simulink model "ABC"  (R2016b)
settings: Solver=VariableStepAuto  StartTime=0.0  StopTime=10.0  RelTol=1e-3
model workspace (MAT data in the model file):
  ContractValidatorBlocksMap = containers.Map
  ContractValidatorBlocksMap.serialization.keys = {'ABC/S/ASpec/validator', 'ABC/S/BSpec/validator', 'ABC/S/CSpec/validator', 'ABC/S_Spec/validator', 'ABC/Subsystem/ASpec/validator', 'ABC/Subsystem/BSpec/validator', 'ABC/Subsystem/BSpec1/validator', 'ABC/contract/validator'}
  ContractValidatorBlocksMap.serialization.values{1}.block = 'ABC/S/ASpec/validator'
  ContractValidatorBlocksMap.serialization.values{1}.assumePorts = 1
  ContractValidatorBlocksMap.serialization.values{1}.guaranteePorts = 1
  ContractValidatorBlocksMap.serialization.values{1}.modeBlocksPorts = 0
  ContractValidatorBlocksMap.serialization.values{1}.portHandles.Inport = [194.002685547 195.002685547]
  ContractValidatorBlocksMap.serialization.values{1}.portHandles.Outport = 196.002685547
  ContractValidatorBlocksMap.serialization.values{1}.portHandles.Enable = []
  ContractValidatorBlocksMap.serialization.values{1}.portHandles.Trigger = []
  ContractValidatorBlocksMap.serialization.values{1}.portHandles.State = []
  ContractValidatorBlocksMap.serialization.values{1}.portHandles.LConn = []
  ContractValidatorBlocksMap.serialization.values{1}.portHandles.RConn = []
  ContractValidatorBlocksMap.serialization.values{1}.portHandles.Ifaction = []
  ContractValidatorBlocksMap.serialization.values{1}.portHandles.Reset = []
  ContractValidatorBlocksMap.serialization.values{1}.portConnectivity(1).Type = '1'
  ContractValidatorBlocksMap.serialization.values{1}.portConnectivity(1).Position = [365 -50]
  ContractValidatorBlocksMap.serialization.values{1}.portConnectivity(1).SrcBlock = 19.0026855469
  ContractValidatorBlocksMap.serialization.values{1}.portConnectivity(1).SrcPort = 0
  ContractValidatorBlocksMap.serialization.values{1}.portConnectivity(1).DstBlock = []
  ContractValidatorBlocksMap.serialization.values{1}.portConnectivity(1).DstPort = []
  ContractValidatorBlocksMap.serialization.values{1}.portConnectivity(2).Type = '2'
  ContractValidatorBlocksMap.serialization.values{1}.portConnectivity(2).Position = [365 200]
  ContractValidatorBlocksMap.serialization.values{1}.portConnectivity(2).SrcBlock = 26.0026855469
  ContractValidatorBlocksMap.serialization.values{1}.portConnectivity(2).SrcPort = 0
  ContractValidatorBlocksMap.serialization.values{1}.portConnectivity(2).DstBlock = []
  ContractValidatorBlocksMap.serialization.values{1}.portConnectivity(2).DstPort = []
  ContractValidatorBlocksMap.serialization.values{1}.portConnectivity(3).Type = '1'
  ContractValidatorBlocksMap.serialization.values{1}.portConnectivity(3).Position = [500 75]
  ContractValidatorBlocksMap.serialization.values{1}.portConnectivity(3).SrcBlock = []
  ContractValidatorBlocksMap.serialization.values{1}.portConnectivity(3).SrcPort = []
  ContractValidatorBlocksMap.serialization.values{1}.portConnectivity(3).DstBlock = 38.0026855469
  ContractValidatorBlocksMap.serialization.values{1}.portConnectivity(3).DstPort = 0
  ContractValidatorBlocksMap.serialization.values{2}.block = 'ABC/S/BSpec/validator'
  ContractValidatorBlocksMap.serialization.values{2}.assumePorts = 1
  ContractValidatorBlocksMap.serialization.values{2}.guaranteePorts = 1
  ContractValidatorBlocksMap.serialization.values{2}.modeBlocksPorts = 0
  ContractValidatorBlocksMap.serialization.values{2}.portHandles.Inport = [191.002685547 192.002685547]
  ContractValidatorBlocksMap.serialization.values{2}.portHandles.Outport = 193.002685547
  ContractValidatorBlocksMap.serialization.values{2}.portHandles.Enable = []
  ContractValidatorBlocksMap.serialization.values{2}.portHandles.Trigger = []
  ContractValidatorBlocksMap.serialization.values{2}.portHandles.State = []
  ContractValidatorBlocksMap.serialization.values{2}.portHandles.LConn = []
  ContractValidatorBlocksMap.serialization.values{2}.portHandles.RConn = []
  ContractValidatorBlocksMap.serialization.values{2}.portHandles.Ifaction = []
  ContractValidatorBlocksMap.serialization.values{2}.portHandles.Reset = []
  ContractValidatorBlocksMap.serialization.values{2}.portConnectivity(1).Type = '1'
  ContractValidatorBlocksMap.serialization.values{2}.portConnectivity(1).Position = [365 -50]
  ContractValidatorBlocksMap.serialization.values{2}.portConnectivity(1).SrcBlock = 60.0026855469
  ContractValidatorBlocksMap.serialization.values{2}.portConnectivity(1).SrcPort = 0
  ContractValidatorBlocksMap.serialization.values{2}.portConnectivity(1).DstBlock = []
  ContractValidatorBlocksMap.serialization.values{2}.portConnectivity(1).DstPort = []
  ContractValidatorBlocksMap.serialization.values{2}.portConnectivity(2).Type = '2'
  ContractValidatorBlocksMap.serialization.values{2}.portConnectivity(2).Position = [365 200]
  ContractValidatorBlocksMap.serialization.values{2}.portConnectivity(2).SrcBlock = 67.0026855469
  ContractValidatorBlocksMap.serialization.values{2}.portConnectivity(2).SrcPort = 0
  ContractValidatorBlocksMap.serialization.values{2}.portConnectivity(2).DstBlock = []
  ContractValidatorBlocksMap.serialization.values{2}.portConnectivity(2).DstPort = []
  ContractValidatorBlocksMap.serialization.values{2}.portConnectivity(3).Type = '1'
  ContractValidatorBlocksMap.serialization.values{2}.portConnectivity(3).Position = [500 75]
  ContractValidatorBlocksMap.serialization.values{2}.portConnectivity(3).SrcBlock = []
  ContractValidatorBlocksMap.serialization.values{2}.portConnectivity(3).SrcPort = []
  ContractValidatorBlocksMap.serialization.values{2}.portConnectivity(3).DstBlock = 81.0026855469
  ContractValidatorBlocksMap.serialization.values{2}.portConnectivity(3).DstPort = 0
  ContractValidatorBlocksMap.serialization.values{3}.block = 'ABC/S/CSpec/validator'
  ContractValidatorBlocksMap.serialization.values{3}.assumePorts = 0
  ContractValidatorBlocksMap.serialization.values{3}.guaranteePorts = 1
  ContractValidatorBlocksMap.serialization.values{3}.modeBlocksPorts = 0
  ContractValidatorBlocksMap.serialization.values{3}.portHandles.Inport = 189.002685547
  ContractValidatorBlocksMap.serialization.values{3}.portHandles.Outport = 190.002685547
  ContractValidatorBlocksMap.serialization.values{3}.portHandles.Enable = []
  ContractValidatorBlocksMap.serialization.values{3}.portHandles.Trigger = []
  ContractValidatorBlocksMap.serialization.values{3}.portHandles.State = []
  ContractValidatorBlocksMap.serialization.values{3}.portHandles.LConn = []
  ContractValidatorBlocksMap.serialization.values{3}.portHandles.RConn = []
  ContractValidatorBlocksMap.serialization.values{3}.portHandles.Ifaction = []
  ContractValidatorBlocksMap.serialization.values{3}.portHandles.Reset = []
  ContractValidatorBlocksMap.serialization.values{3}.portConnectivity(1).Type = '1'
  ContractValidatorBlocksMap.serialization.values{3}.portConnectivity(1).Position = [365 110]
  ContractValidatorBlocksMap.serialization.values{3}.portConnectivity(1).SrcBlock = 104.002685547
  ContractValidatorBlocksMap.serialization.values{3}.portConnectivity(1).SrcPort = 0
  ContractValidatorBlocksMap.serialization.values{3}.portConnectivity(1).DstBlock = []
  ContractValidatorBlocksMap.serialization.values{3}.portConnectivity(1).DstPort = []
  ContractValidatorBlocksMap.serialization.values{3}.portConnectivity(2).Type = '1'
  ContractValidatorBlocksMap.serialization.values{3}.portConnectivity(2).Position = [465 110]
  ContractValidatorBlocksMap.serialization.values{3}.portConnectivity(2).SrcBlock = []
  ContractValidatorBlocksMap.serialization.values{3}.portConnectivity(2).SrcPort = []
  ContractValidatorBlocksMap.serialization.values{3}.portConnectivity(2).DstBlock = 118.002685547
  ContractValidatorBlocksMap.serialization.values{3}.portConnectivity(2).DstPort = 0
  ContractValidatorBlocksMap.serialization.values{4}.block = 'ABC/S_Spec/validator'
  ContractValidatorBlocksMap.serialization.values{4}.assumePorts = 1
  ContractValidatorBlocksMap.serialization.values{4}.guaranteePorts = 1
  ContractValidatorBlocksMap.serialization.values{4}.modeBlocksPorts = 0
  ContractValidatorBlocksMap.serialization.values{4}.portHandles.Inport = [186.002685547 187.002685547]
  ContractValidatorBlocksMap.serialization.values{4}.portHandles.Outport = 188.002685547
  ContractValidatorBlocksMap.serialization.values{4}.portHandles.Enable = []
  ContractValidatorBlocksMap.serialization.values{4}.portHandles.Trigger = []
  ContractValidatorBlocksMap.serialization.values{4}.portHandles.State = []
  ContractValidatorBlocksMap.serialization.values{4}.portHandles.LConn = []
  ContractValidatorBlocksMap.serialization.values{4}.portHandles.RConn = []
  ContractValidatorBlocksMap.serialization.values{4}.portHandles.Ifaction = []
  ContractValidatorBlocksMap.serialization.values{4}.portHandles.Reset = []
  ContractValidatorBlocksMap.serialization.values{4}.portConnectivity(1).Type = '1'
  ContractValidatorBlocksMap.serialization.values{4}.portConnectivity(1).Position = [365 -50]
  ContractValidatorBlocksMap.serialization.values{4}.portConnectivity(1).SrcBlock = 154.002685547
  ContractValidatorBlocksMap.serialization.values{4}.portConnectivity(1).SrcPort = 0
  ContractValidatorBlocksMap.serialization.values{4}.portConnectivity(1).DstBlock = []
  ContractValidatorBlocksMap.serialization.values{4}.portConnectivity(1).DstPort = []
  ContractValidatorBlocksMap.serialization.values{4}.portConnectivity(2).Type = '2'
  ContractValidatorBlocksMap.serialization.values{4}.portConnectivity(2).Position = [365 200]
  ContractValidatorBlocksMap.serialization.values{4}.portConnectivity(2).SrcBlock = 161.002685547
  ContractValidatorBlocksMap.serialization.values{4}.portConnectivity(2).SrcPort = 0
  ContractValidatorBlocksMap.serialization.values{4}.portConnectivity(2).DstBlock = []
  ContractValidatorBlocksMap.serialization.values{4}.portConnectivity(2).DstPort = []
  ContractValidatorBlocksMap.serialization.values{4}.portConnectivity(3).Type = '1'
  ContractValidatorBlocksMap.serialization.values{4}.portConnectivity(3).Position = [500 75]
  ContractValidatorBlocksMap.serialization.values{4}.portConnectivity(3).SrcBlock = []
  ContractValidatorBlocksMap.serialization.values{4}.portConnectivity(3).SrcPort = []
  ContractValidatorBlocksMap.serialization.values{4}.portConnectivity(3).DstBlock = 169.002685547
  ContractValidatorBlocksMap.serialization.values{4}.portConnectivity(3).DstPort = 0
  ContractValidatorBlocksMap.serialization.values{5}.block = 'ABC/Subsystem/ASpec/validator'
  ContractValidatorBlocksMap.serialization.values{5}.assumePorts = 1
  ContractValidatorBlocksMap.serialization.values{5}.guaranteePorts = 1
  ContractValidatorBlocksMap.serialization.values{5}.modeBlocksPorts = 0
  ContractValidatorBlocksMap.serialization.values{5}.portHandles.Inport = [529.000610352 530.000610352]
  ContractValidatorBlocksMap.serialization.values{5}.portHandles.Outport = 531.000610352
  ContractValidatorBlocksMap.serialization.values{5}.portHandles.Enable = []
  ContractValidatorBlocksMap.serialization.values{5}.portHandles.Trigger = []
  ContractValidatorBlocksMap.serialization.values{5}.portHandles.State = []
  ContractValidatorBlocksMap.serialization.values{5}.portHandles.LConn = []
  ContractValidatorBlocksMap.serialization.values{5}.portHandles.RConn = []
  ContractValidatorBlocksMap.serialization.values{5}.portHandles.Ifaction = []
  ContractValidatorBlocksMap.serialization.values{5}.portHandles.Reset = []
  ContractValidatorBlocksMap.serialization.values{5}.portConnectivity(1).Type = '1'
  ContractValidatorBlocksMap.serialization.values{5}.portConnectivity(1).Position = [365 -50]
  ContractValidatorBlocksMap.serialization.values{5}.portConnectivity(1).SrcBlock = 305.000732422
  ContractValidatorBlocksMap.serialization.values{5}.portConnectivity(1).SrcPort = 0
  ContractValidatorBlocksMap.serialization.values{5}.portConnectivity(1).DstBlock = []
  ContractValidatorBlocksMap.serialization.values{5}.portConnectivity(1).DstPort = []
  ContractValidatorBlocksMap.serialization.values{5}.portConnectivity(2).Type = '2'
  ContractValidatorBlocksMap.serialization.values{5}.portConnectivity(2).Position = [365 200]
  ContractValidatorBlocksMap.serialization.values{5}.portConnectivity(2).SrcBlock = 319.000732422
  ContractValidatorBlocksMap.serialization.values{5}.portConnectivity(2).SrcPort = 0
  ContractValidatorBlocksMap.serialization.values{5}.portConnectivity(2).DstBlock = []
  ContractValidatorBlocksMap.serialization.values{5}.portConnectivity(2).DstPort = []
  ContractValidatorBlocksMap.serialization.values{5}.portConnectivity(3).Type = '1'
  ContractValidatorBlocksMap.serialization.values{5}.portConnectivity(3).Position = [500 75]
  ContractValidatorBlocksMap.serialization.values{5}.portConnectivity(3).SrcBlock = []
  ContractValidatorBlocksMap.serialization.values{5}.portConnectivity(3).SrcPort = []
  ContractValidatorBlocksMap.serialization.values{5}.portConnectivity(3).DstBlock = 351.000610352
  ContractValidatorBlocksMap.serialization.values{5}.portConnectivity(3).DstPort = 0
  ContractValidatorBlocksMap.serialization.values{6}.block = 'ABC/Subsystem/BSpec/validator'
  ContractValidatorBlocksMap.serialization.values{6}.assumePorts = 1
  ContractValidatorBlocksMap.serialization.values{6}.guaranteePorts = 1
  ContractValidatorBlocksMap.serialization.values{6}.modeBlocksPorts = 0
  ContractValidatorBlocksMap.serialization.values{6}.portHandles.Inport = [523.000610352 525.000610352]
  ContractValidatorBlocksMap.serialization.values{6}.portHandles.Outport = 526.000610352
  ContractValidatorBlocksMap.serialization.values{6}.portHandles.Enable = []
  ContractValidatorBlocksMap.serialization.values{6}.portHandles.Trigger = []
  ContractValidatorBlocksMap.serialization.values{6}.portHandles.State = []
  ContractValidatorBlocksMap.serialization.values{6}.portHandles.LConn = []
  ContractValidatorBlocksMap.serialization.values{6}.portHandles.RConn = []
  ContractValidatorBlocksMap.serialization.values{6}.portHandles.Ifaction = []
  ContractValidatorBlocksMap.serialization.values{6}.portHandles.Reset = []
  ContractValidatorBlocksMap.serialization.values{6}.portConnectivity(1).Type = '1'
  ContractValidatorBlocksMap.serialization.values{6}.portConnectivity(1).Position = [365 -50]
  ContractValidatorBlocksMap.serialization.values{6}.portConnectivity(1).SrcBlock = 378.000610352
  ContractValidatorBlocksMap.serialization.values{6}.portConnectivity(1).SrcPort = 0
  ContractValidatorBlocksMap.serialization.values{6}.portConnectivity(1).DstBlock = []
  ContractValidatorBlocksMap.serialization.values{6}.portConnectivity(1).DstPort = []
  ContractValidatorBlocksMap.serialization.values{6}.portConnectivity(2).Type = '2'
  ContractValidatorBlocksMap.serialization.values{6}.portConnectivity(2).Position = [365 200]
  ContractValidatorBlocksMap.serialization.values{6}.portConnectivity(2).SrcBlock = 384.000610352
  ContractValidatorBlocksMap.serialization.values{6}.portConnectivity(2).SrcPort = 0
  ContractValidatorBlocksMap.serialization.values{6}.portConnectivity(2).DstBlock = []
  ContractValidatorBlocksMap.serialization.values{6}.portConnectivity(2).DstPort = []
  ContractValidatorBlocksMap.serialization.values{6}.portConnectivity(3).Type = '1'
  ContractValidatorBlocksMap.serialization.values{6}.portConnectivity(3).Position = [500 75]
  ContractValidatorBlocksMap.serialization.values{6}.portConnectivity(3).SrcBlock = []
  ContractValidatorBlocksMap.serialization.values{6}.portConnectivity(3).SrcPort = []
  ContractValidatorBlocksMap.serialization.values{6}.portConnectivity(3).DstBlock = 401.000610352
  ContractValidatorBlocksMap.serialization.values{6}.portConnectivity(3).DstPort = 0
  ContractValidatorBlocksMap.serialization.values{7}.block = 'ABC/Subsystem/BSpec1/validator'
  ContractValidatorBlocksMap.serialization.values{7}.assumePorts = 0
  ContractValidatorBlocksMap.serialization.values{7}.guaranteePorts = 1
  ContractValidatorBlocksMap.serialization.values{7}.modeBlocksPorts = 0
  ContractValidatorBlocksMap.serialization.values{7}.portHandles.Inport = 527.000610352
  ContractValidatorBlocksMap.serialization.values{7}.portHandles.Outport = 528.000610352
  ContractValidatorBlocksMap.serialization.values{7}.portHandles.Enable = []
  ContractValidatorBlocksMap.serialization.values{7}.portHandles.Trigger = []
  ContractValidatorBlocksMap.serialization.values{7}.portHandles.State = []
  ContractValidatorBlocksMap.serialization.values{7}.portHandles.LConn = []
  ContractValidatorBlocksMap.serialization.values{7}.portHandles.RConn = []
  ContractValidatorBlocksMap.serialization.values{7}.portHandles.Ifaction = []
  ContractValidatorBlocksMap.serialization.values{7}.portHandles.Reset = []
  ContractValidatorBlocksMap.serialization.values{7}.portConnectivity(1).Type = '1'
  ContractValidatorBlocksMap.serialization.values{7}.portConnectivity(1).Position = [365 110]
  ContractValidatorBlocksMap.serialization.values{7}.portConnectivity(1).SrcBlock = 417.000610352
  ContractValidatorBlocksMap.serialization.values{7}.portConnectivity(1).SrcPort = 0
  ContractValidatorBlocksMap.serialization.values{7}.portConnectivity(1).DstBlock = []
  ContractValidatorBlocksMap.serialization.values{7}.portConnectivity(1).DstPort = []
  ContractValidatorBlocksMap.serialization.values{7}.portConnectivity(2).Type = '1'
  ContractValidatorBlocksMap.serialization.values{7}.portConnectivity(2).Position = [465 110]
  ContractValidatorBlocksMap.serialization.values{7}.portConnectivity(2).SrcBlock = []
  ContractValidatorBlocksMap.serialization.values{7}.portConnectivity(2).SrcPort = []
  ContractValidatorBlocksMap.serialization.values{7}.portConnectivity(2).DstBlock = 430.000610352
  ContractValidatorBlocksMap.serialization.values{7}.portConnectivity(2).DstPort = 0
  ContractValidatorBlocksMap.serialization.values{8}.block = 'ABC/contract/validator'
  ContractValidatorBlocksMap.serialization.values{8}.assumePorts = 1
  ContractValidatorBlocksMap.serialization.values{8}.guaranteePorts = 1
  ContractValidatorBlocksMap.serialization.values{8}.modeBlocksPorts = 0
  ContractValidatorBlocksMap.serialization.values{8}.portHandles.Inport = [507.000610352 521.000610352]
  ContractValidatorBlocksMap.serialization.values{8}.portHandles.Outport = 522.000610352
  ContractValidatorBlocksMap.serialization.values{8}.portHandles.Enable = []
  ContractValidatorBlocksMap.serialization.values{8}.portHandles.Trigger = []
  ContractValidatorBlocksMap.serialization.values{8}.portHandles.State = []
  ContractValidatorBlocksMap.serialization.values{8}.portHandles.LConn = []
  ContractValidatorBlocksMap.serialization.values{8}.portHandles.RConn = []
  ContractValidatorBlocksMap.serialization.values{8}.portHandles.Ifaction = []
  ContractValidatorBlocksMap.serialization.values{8}.portHandles.Reset = []
  ContractValidatorBlocksMap.serialization.values{8}.portConnectivity(1).Type = '1'
  ContractValidatorBlocksMap.serialization.values{8}.portConnectivity(1).Position = [365 -50]
  ContractValidatorBlocksMap.serialization.values{8}.portConnectivity(1).SrcBlock = 472.000610352
  ContractValidatorBlocksMap.serialization.values{8}.portConnectivity(1).SrcPort = 0
  ContractValidatorBlocksMap.serialization.values{8}.portConnectivity(1).DstBlock = []
  ContractValidatorBlocksMap.serialization.values{8}.portConnectivity(1).DstPort = []
  ContractValidatorBlocksMap.serialization.values{8}.portConnectivity(2).Type = '2'
  ContractValidatorBlocksMap.serialization.values{8}.portConnectivity(2).Position = [365 200]
  ContractValidatorBlocksMap.serialization.values{8}.portConnectivity(2).SrcBlock = 478.000610352
  ContractValidatorBlocksMap.serialization.values{8}.portConnectivity(2).SrcPort = 0
  ContractValidatorBlocksMap.serialization.values{8}.portConnectivity(2).DstBlock = []
  ContractValidatorBlocksMap.serialization.values{8}.portConnectivity(2).DstPort = []
  ContractValidatorBlocksMap.serialization.values{8}.portConnectivity(3).Type = '1'
  ContractValidatorBlocksMap.serialization.values{8}.portConnectivity(3).Position = [500 75]
  ContractValidatorBlocksMap.serialization.values{8}.portConnectivity(3).SrcBlock = []
  ContractValidatorBlocksMap.serialization.values{8}.portConnectivity(3).SrcPort = []
  ContractValidatorBlocksMap.serialization.values{8}.portConnectivity(3).DstBlock = 485.000610352
  ContractValidatorBlocksMap.serialization.values{8}.portConnectivity(3).DstPort = 0
  ContractValidatorBlocksMap.serialization.uniformity = 0
  ContractValidatorBlocksMap.serialization.keyType = 'char'
  ContractValidatorBlocksMap.serialization.valueType = 'any'
undefined symbols (not defined in the file): contractAfterSimulation, ContractAssumeBlock, contractBeforeSimulation, ContractBlock, ContractGuaranteeBlock, ContractValidatorBlock, saveValidatorParameters
libraries: simulink x4
settings Model: Creator=hbourbou  LastModifiedBy=hbourbou
settings DataIOCC: ReturnWorkspaceOutputs=on
settings SFSimCC: SimUseLocalCustomCode=on
settings RTWCC: RTWUseLocalCustomCode=on

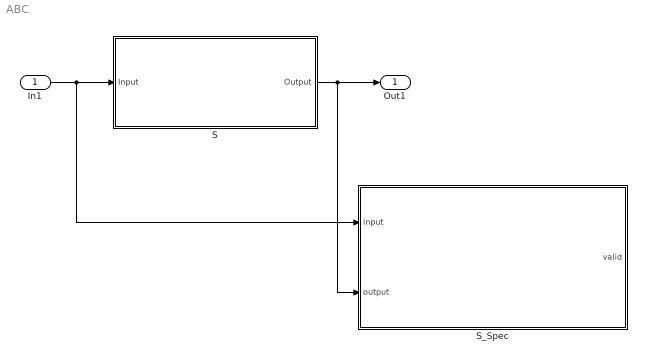
== system ABC ==
  In1 : Inport  OutDataTypeStr=int8
  S : Subsystem
  S_Spec : Subsystem  mask(ContractBlock){ContractBlockType=ContractBlock}
      mask init:
      | set_param(gcb, 'LinkStatus', 'none');
      settings: CopyFcn=set_param(gcb, 'LinkStatus', 'none');
      mask DialogControl DescTextVar Prompt: Contract block
      mask Display:
      | text(0.5, 0.5, '{\bf\fontsize{20}Contract}', 'hor', 'center', 'texmode','on');
      | blocks = find_system(gcb, 'LookUnderMasks','all', 'SearchDepth',1,'BlockType','Inport');
      | for i = 1 : length(blocks)
      |     blockName = get_param(blocks(i), 'Name');
      |     [path, blockName] = fileparts(char(blockName));
      |     port_label('input', i, blockName);
      | end
      | 
      | blocks = find_system(gcb, 'LookUnderMasks','all', 'SearchDepth',1,'BlockType','Outport');
      | for i = 1 : length(blocks)
      |     blockName = get_param(blocks(i), 'Name');
      |     [path, blockName] = fileparts(char(blockName));
      |     port_label('output', i, blockName);
      | end
  Out1 : Outport
  wires:
  In1/1 -> S_Spec/1(input), S/1(Input)
  S/1(Output) -> S_Spec/2(output), Out1/1

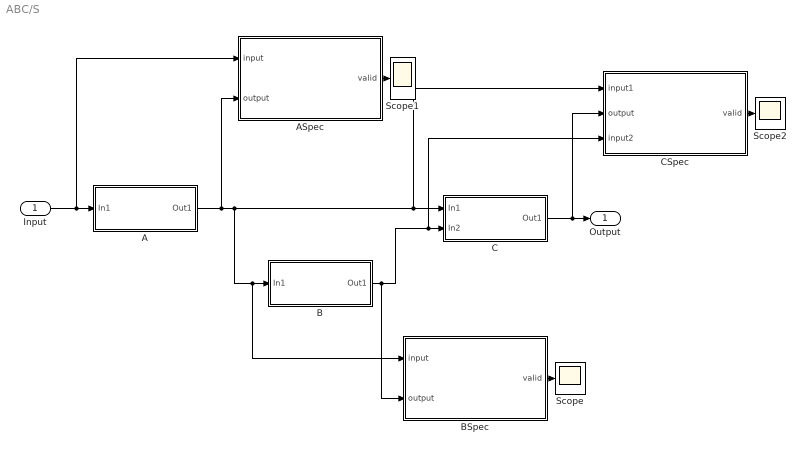
== system ABC/S ==
  Input : Inport
  A : Subsystem
  ASpec : Subsystem  mask(ContractBlock){ContractBlockType=ContractBlock}
      mask init:
      | set_param(gcb, 'LinkStatus', 'none');
      settings: CopyFcn=set_param(gcb, 'LinkStatus', 'none');
      mask DialogControl DescTextVar Prompt: Contract block
      mask Display:
      | text(0.5, 0.5, '{\bf\fontsize{20}Contract}', 'hor', 'center', 'texmode','on');
      | blocks = find_system(gcb, 'LookUnderMasks','all', 'SearchDepth',1,'BlockType','Inport');
      | for i = 1 : length(blocks)
      |     blockName = get_param(blocks(i), 'Name');
      |     [path, blockName] = fileparts(char(blockName));
      |     port_label('input', i, blockName);
      | end
      | 
      | blocks = find_system(gcb, 'LookUnderMasks','all', 'SearchDepth',1,'BlockType','Outport');
      | for i = 1 : length(blocks)
      |     blockName = get_param(blocks(i), 'Name');
      |     [path, blockName] = fileparts(char(blockName));
      |     port_label('output', i, blockName);
      | end
  B : Subsystem
  BSpec : Subsystem  mask(ContractBlock){ContractBlockType=ContractBlock}
      mask init:
      | set_param(gcb, 'LinkStatus', 'none');
      settings: CopyFcn=set_param(gcb, 'LinkStatus', 'none');
      mask DialogControl DescTextVar Prompt: Contract block
      mask Display:
      | text(0.5, 0.5, '{\bf\fontsize{20}Contract}', 'hor', 'center', 'texmode','on');
      | blocks = find_system(gcb, 'LookUnderMasks','all', 'SearchDepth',1,'BlockType','Inport');
      | for i = 1 : length(blocks)
      |     blockName = get_param(blocks(i), 'Name');
      |     [path, blockName] = fileparts(char(blockName));
      |     port_label('input', i, blockName);
      | end
      | 
      | blocks = find_system(gcb, 'LookUnderMasks','all', 'SearchDepth',1,'BlockType','Outport');
      | for i = 1 : length(blocks)
      |     blockName = get_param(blocks(i), 'Name');
      |     [path, blockName] = fileparts(char(blockName));
      |     port_label('output', i, blockName);
      | end
  C : Subsystem
  CSpec : Subsystem  mask(ContractBlock){ContractBlockType=ContractBlock}
      mask init:
      | set_param(gcb, 'LinkStatus', 'none');
      settings: CopyFcn=set_param(gcb, 'LinkStatus', 'none');
      mask DialogControl DescTextVar Prompt: Contract block
      mask Display:
      | text(0.5, 0.5, '{\bf\fontsize{20}Contract}', 'hor', 'center', 'texmode','on');
      | blocks = find_system(gcb, 'LookUnderMasks','all', 'SearchDepth',1,'BlockType','Inport');
      | for i = 1 : length(blocks)
      |     blockName = get_param(blocks(i), 'Name');
      |     [path, blockName] = fileparts(char(blockName));
      |     port_label('input', i, blockName);
      | end
      | 
      | blocks = find_system(gcb, 'LookUnderMasks','all', 'SearchDepth',1,'BlockType','Outport');
      | for i = 1 : length(blocks)
      |     blockName = get_param(blocks(i), 'Name');
      |     [path, blockName] = fileparts(char(blockName));
      |     port_label('output', i, blockName);
      | end
  Scope : Scope
  Scope1 : Scope
  Scope2 : Scope
  Output : Outport
  wires:
  Input/1 -> ASpec/1(input), A/1(In1)
  C/1(Out1) -> CSpec/2(output), Output/1
  B/1(Out1) -> BSpec/2(output), CSpec/3(input2), C/2(In2)
  A/1(Out1) -> ASpec/2(output), BSpec/1(input), B/1(In1), CSpec/1(input1), C/1(In1)
  BSpec/1(valid) -> Scope/1
  ASpec/1(valid) -> Scope1/1
  CSpec/1(valid) -> Scope2/1

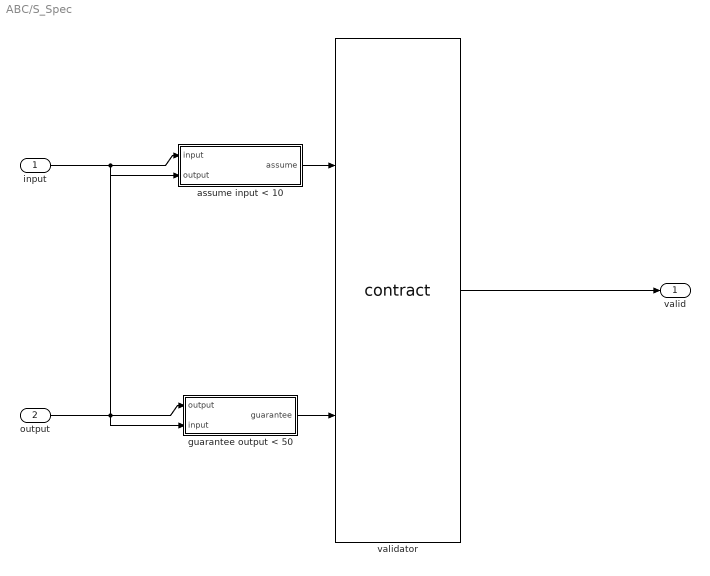
== system ABC/S_Spec ==
  input : Inport
  output : Inport  Port=2
  assume input < 10 : Subsystem  mask(ContractAssumeBlock){ContractBlockType=ContractAssumeBlock}
      mask init:
      | set_param(gcb, 'LinkStatus', 'none');
      mask DialogControl DescTextVar Prompt: Assume block
  guarantee output < 50 : Subsystem  mask(ContractGuaranteeBlock){ContractBlockType=ContractGuaranteeBlock}
      mask init:
      | set_param(gcb, 'LinkStatus', 'none');
      mask DialogControl DescTextVar Prompt: Guarantee block
  validator : M-S-Function  LoadFcn=saveValidatorParameters(gcb);  InitFcn=contractBeforeSimulation();  StopFcn=contractAfterSimulation();  FunctionName=contract  mask(ContractValidatorBlock){assumePorts=1, guaranteePorts=1, modePorts=0, ContractBlockType=ContractValidatorBlock, createInportsCheckbox=on}
      mask prompts: assumePorts "Assume ports     :"; guaranteePorts "Guarantee ports :"; modePorts "Mode ports        :"; createInportsCheckbox "Create inports and connect them automatically"
      mask init:
      | set_param(gcb,'LinkStatus','none');
      | contract_callback('inputs_callback',gcb);
      mask DialogControl DescTextVar Prompt: The validator block implements the following logic: <br> <br> <b>Sofar</b>(assume<sub>1</sub> <b>&#8743;</b> assume<sub>2</sub> <b>&#8743;</b> ... assume<sub>k</sub>) <b>&rarr;</b> (guarantee<sub>1</sub> <b>&#8743;</b> guarantee<sub>2</sub> <b>&#8743;</b> ... guarantee<sub>m</sub> <b>&#8743;</b>  mode<sub>1</sub> <b>&#8743;</b> mode<sub>2</sub> <b>&#8743;</b> ... <b>&#8743;</b> mode<sub>n</sub> )<br> where mode<sub>i</sub> = require<sub>i</sub> <b>&rarr;</b> ensure<sub>i</sub>
      mask Display:
      | color('black');
      | port_label('input',1,'assume');
      | port_label('input',2,'guarantee');
      | port_label('output',1,'valid');
  valid : Outport
  wires:
  output/1 -> guarantee output < 50/1(output), assume input < 10/2(output)
  input/1 -> assume input < 10/1(input), guarantee output < 50/2(input)
  validator/1 -> valid/1
  assume input < 10/1(assume) -> validator/1
  guarantee output < 50/1(guarantee) -> validator/2

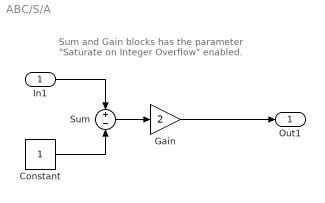
== system ABC/S/A ==
  note: Sum and Gain blocks has the parameter
      | "Saturate on Integer Overflow" enabled.
  In1 : Inport
  Constant : Constant  OutDataTypeStr=Inherit: Inherit via back propagation
  Gain : Gain  Gain=2  OutDataTypeStr=Inherit: Inherit via back propagation  SaturateOnIntegerOverflow=on  ParamDataTypeStr=Inherit: Same as input
  Sum : Sum  Inputs=+-  SaturateOnIntegerOverflow=on
  Out1 : Outport
  wires:
  In1/1 -> Sum/1
  Gain/1 -> Out1/1
  Sum/1 -> Gain/1
  Constant/1 -> Sum/2

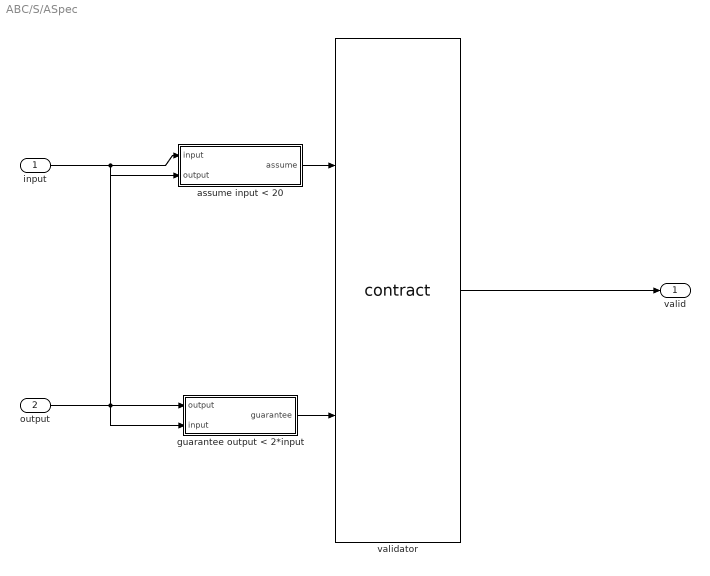
== system ABC/S/ASpec ==
  input : Inport
  output : Inport  Port=2
  assume input < 20 : Subsystem  mask(ContractAssumeBlock){ContractBlockType=ContractAssumeBlock}
      mask init:
      | set_param(gcb, 'LinkStatus', 'none');
      mask DialogControl DescTextVar Prompt: Assume block
  guarantee output < 2*input : Subsystem  mask(ContractGuaranteeBlock){ContractBlockType=ContractGuaranteeBlock}
      mask init:
      | set_param(gcb, 'LinkStatus', 'none');
      mask DialogControl DescTextVar Prompt: Guarantee block
  validator : M-S-Function  LoadFcn=saveValidatorParameters(gcb);  InitFcn=contractBeforeSimulation();  StopFcn=contractAfterSimulation();  FunctionName=contract  mask(ContractValidatorBlock){assumePorts=1, guaranteePorts=1, modePorts=0, ContractBlockType=ContractValidatorBlock, createInportsCheckbox=on}
      mask prompts: assumePorts "Assume ports     :"; guaranteePorts "Guarantee ports :"; modePorts "Mode ports        :"; createInportsCheckbox "Create inports and connect them automatically"
      mask init:
      | set_param(gcb,'LinkStatus','none');
      | contract_callback('inputs_callback',gcb);
      mask DialogControl DescTextVar Prompt: The validator block implements the following logic: <br> <br> <b>Sofar</b>(assume<sub>1</sub> <b>&#8743;</b> assume<sub>2</sub> <b>&#8743;</b> ... assume<sub>k</sub>) <b>&rarr;</b> (guarantee<sub>1</sub> <b>&#8743;</b> guarantee<sub>2</sub> <b>&#8743;</b> ... guarantee<sub>m</sub> <b>&#8743;</b>  mode<sub>1</sub> <b>&#8743;</b> mode<sub>2</sub> <b>&#8743;</b> ... <b>&#8743;</b> mode<sub>n</sub> )<br> where mode<sub>i</sub> = require<sub>i</sub> <b>&rarr;</b> ensure<sub>i</sub>
      mask Display:
      | color('black');
      | port_label('input',1,'assume');
      | port_label('input',2,'guarantee');
      | port_label('output',1,'valid');
  valid : Outport
  wires:
  output/1 -> guarantee output < 2*input/1(output), assume input < 20/2(output)
  input/1 -> assume input < 20/1(input), guarantee output < 2*input/2(input)
  validator/1 -> valid/1
  assume input < 20/1(assume) -> validator/1
  guarantee output < 2*input/1(guarantee) -> validator/2

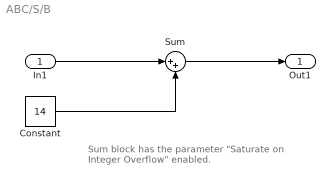
== system ABC/S/B ==
  note: Sum block has the parameter
      | "Saturate on Integer Overflow" enabled.
  In1 : Inport
  Constant : Constant  Value=14  OutDataTypeStr=Inherit: Inherit via back propagation
  Sum : Sum  Inputs=|++  SaturateOnIntegerOverflow=on
  Out1 : Outport
  wires:
  In1/1 -> Sum/1
  Sum/1 -> Out1/1
  Constant/1 -> Sum/2

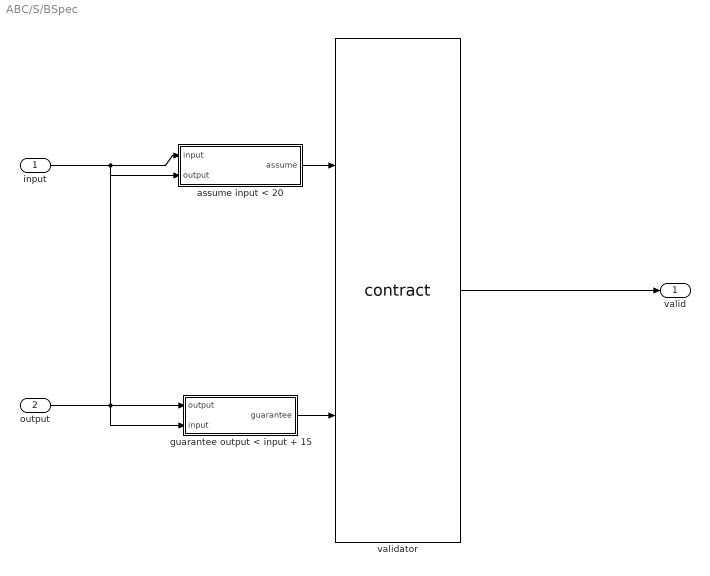
== system ABC/S/BSpec ==
  input : Inport
  output : Inport  Port=2
  assume input < 20 : Subsystem  mask(ContractAssumeBlock){ContractBlockType=ContractAssumeBlock}
      mask init:
      | set_param(gcb, 'LinkStatus', 'none');
      mask DialogControl DescTextVar Prompt: Assume block
  guarantee output < input + 15 : Subsystem  mask(ContractGuaranteeBlock){ContractBlockType=ContractGuaranteeBlock}
      mask init:
      | set_param(gcb, 'LinkStatus', 'none');
      mask DialogControl DescTextVar Prompt: Guarantee block
  validator : M-S-Function  LoadFcn=saveValidatorParameters(gcb);  InitFcn=contractBeforeSimulation();  StopFcn=contractAfterSimulation();  FunctionName=contract  mask(ContractValidatorBlock){assumePorts=1, guaranteePorts=1, modePorts=0, ContractBlockType=ContractValidatorBlock, createInportsCheckbox=on}
      mask prompts: assumePorts "Assume ports     :"; guaranteePorts "Guarantee ports :"; modePorts "Mode ports        :"; createInportsCheckbox "Create inports and connect them automatically"
      mask init:
      | set_param(gcb,'LinkStatus','none');
      | contract_callback('inputs_callback',gcb);
      mask DialogControl DescTextVar Prompt: The validator block implements the following logic: <br> <br> <b>Sofar</b>(assume<sub>1</sub> <b>&#8743;</b> assume<sub>2</sub> <b>&#8743;</b> ... assume<sub>k</sub>) <b>&rarr;</b> (guarantee<sub>1</sub> <b>&#8743;</b> guarantee<sub>2</sub> <b>&#8743;</b> ... guarantee<sub>m</sub> <b>&#8743;</b>  mode<sub>1</sub> <b>&#8743;</b> mode<sub>2</sub> <b>&#8743;</b> ... <b>&#8743;</b> mode<sub>n</sub> )<br> where mode<sub>i</sub> = require<sub>i</sub> <b>&rarr;</b> ensure<sub>i</sub>
      mask Display:
      | color('black');
      | port_label('input',1,'assume');
      | port_label('input',2,'guarantee');
      | port_label('output',1,'valid');
  valid : Outport
  wires:
  output/1 -> guarantee output < input + 15/1(output), assume input < 20/2(output)
  input/1 -> assume input < 20/1(input), guarantee output < input + 15/2(input)
  validator/1 -> valid/1
  assume input < 20/1(assume) -> validator/1
  guarantee output < input + 15/1(guarantee) -> validator/2

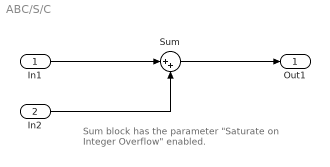
== system ABC/S/C ==
  note: Sum block has the parameter
      | "Saturate on Integer Overflow" enabled.
  In1 : Inport
  In2 : Inport  Port=2
  Sum : Sum  Inputs=|++  SaturateOnIntegerOverflow=on
  Out1 : Outport
  wires:
  In1/1 -> Sum/1
  Sum/1 -> Out1/1
  In2/1 -> Sum/2

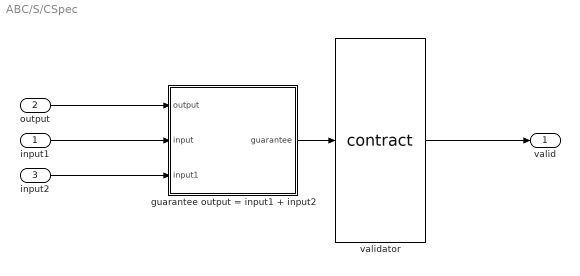
== system ABC/S/CSpec ==
  input1 : Inport
  output : Inport  Port=2
  input2 : Inport  Port=3
  guarantee output = input1 + input2 : Subsystem  mask(ContractGuaranteeBlock){ContractBlockType=ContractGuaranteeBlock}
      mask init:
      | set_param(gcb, 'LinkStatus', 'none');
      mask DialogControl DescTextVar Prompt: Guarantee block
  validator : M-S-Function  LoadFcn=saveValidatorParameters(gcb);  InitFcn=contractBeforeSimulation();  StopFcn=contractAfterSimulation();  FunctionName=contract  mask(ContractValidatorBlock){assumePorts=0, guaranteePorts=1, modePorts=0, ContractBlockType=ContractValidatorBlock, createInportsCheckbox=on}
      mask prompts: assumePorts "Assume ports     :"; guaranteePorts "Guarantee ports :"; modePorts "Mode ports        :"; createInportsCheckbox "Create inports and connect them automatically"
      mask init:
      | set_param(gcb,'LinkStatus','none');
      | contract_callback('inputs_callback',gcb);
      mask DialogControl DescTextVar Prompt: The validator block implements the following logic: <br> <br> <b>Sofar</b>(assume<sub>1</sub> <b>&#8743;</b> assume<sub>2</sub> <b>&#8743;</b> ... assume<sub>k</sub>) <b>&rarr;</b> (guarantee<sub>1</sub> <b>&#8743;</b> guarantee<sub>2</sub> <b>&#8743;</b> ... guarantee<sub>m</sub> <b>&#8743;</b>  mode<sub>1</sub> <b>&#8743;</b> mode<sub>2</sub> <b>&#8743;</b> ... <b>&#8743;</b> mode<sub>n</sub> )<br> where mode<sub>i</sub> = require<sub>i</sub> <b>&rarr;</b> ensure<sub>i</sub>
      mask Display:
      | color('black');
      | port_label('input',1,'guarantee');
      | port_label('output',1,'valid');
  valid : Outport
  wires:
  output/1 -> guarantee output = input1 + input2/1(output)
  validator/1 -> valid/1
  guarantee output = input1 + input2/1(guarantee) -> validator/1
  input1/1 -> guarantee output = input1 + input2/2(input)
  input2/1 -> guarantee output = input1 + input2/3(input1)

== system ABC/S_Spec/assume input < 10 ==
  input : Inport
  output : Inport  Port=2
  Compare To Constant : simulink/Logic and Bit Operations/Compare To Constant  relop=<  const=10  OutDataTypeStr=boolean
  assume : Outport  OutDataTypeStr=boolean
  wires:
  Compare To Constant/1 -> assume/1
  input/1 -> Compare To Constant/1

== system ABC/S_Spec/guarantee output < 50 ==
  output : Inport
  input : Inport  Port=2
  Compare To Constant : simulink/Logic and Bit Operations/Compare To Constant  relop=<  const=50  OutDataTypeStr=boolean
  guarantee : Outport  OutDataTypeStr=boolean
  wires:
  Compare To Constant/1 -> guarantee/1
  output/1 -> Compare To Constant/1

== system ABC/S/ASpec/assume input < 20 ==
  input : Inport
  output : Inport  Port=2
  Compare To Constant : simulink/Logic and Bit Operations/Compare To Constant  relop=<  const=20  OutDataTypeStr=boolean
  assume : Outport  OutDataTypeStr=boolean
  wires:
  Compare To Constant/1 -> assume/1
  input/1 -> Compare To Constant/1

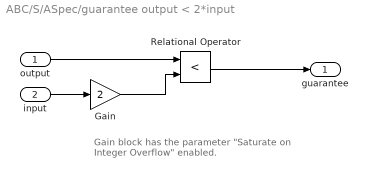
== system ABC/S/ASpec/guarantee output < 2*input ==
  note: Gain block has the parameter
      | "Saturate on Integer Overflow" enabled.
  output : Inport
  input : Inport  Port=2
  Gain : Gain  Gain=2  OutDataTypeStr=int8  SaturateOnIntegerOverflow=on
  Relational Operator : RelationalOperator  Operator=<  OutDataTypeStr=boolean  RndMeth=Simplest
  guarantee : Outport  OutDataTypeStr=boolean
  wires:
  Relational Operator/1 -> guarantee/1
  output/1 -> Relational Operator/1
  input/1 -> Gain/1
  Gain/1 -> Relational Operator/2

== system ABC/S/BSpec/assume input < 20 ==
  input : Inport
  output : Inport  Port=2
  Compare To Constant : simulink/Logic and Bit Operations/Compare To Constant  relop=<  const=20  OutDataTypeStr=boolean
  assume : Outport  OutDataTypeStr=boolean
  wires:
  Compare To Constant/1 -> assume/1
  input/1 -> Compare To Constant/1

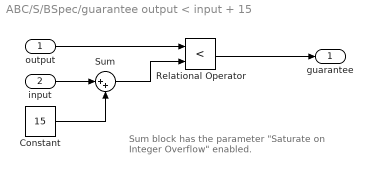
== system ABC/S/BSpec/guarantee output < input + 15 ==
  note: Sum block has the parameter
      | "Saturate on Integer Overflow" enabled.
  output : Inport
  input : Inport  Port=2
  Constant : Constant  Value=15
  Relational Operator : RelationalOperator  Operator=<  OutDataTypeStr=boolean  RndMeth=Simplest
  Sum : Sum  Inputs=|++  SaturateOnIntegerOverflow=on
  guarantee : Outport  OutDataTypeStr=boolean
  wires:
  Relational Operator/1 -> guarantee/1
  output/1 -> Relational Operator/1
  input/1 -> Sum/1
  Sum/1 -> Relational Operator/2
  Constant/1 -> Sum/2

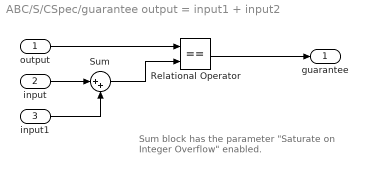
== system ABC/S/CSpec/guarantee output = input1 + input2 ==
  note: Sum block has the parameter
      | "Saturate on Integer Overflow" enabled.
  output : Inport
  input : Inport  Port=2
  input1 : Inport  Port=3
  Relational Operator : RelationalOperator  Operator===  OutDataTypeStr=boolean  RndMeth=Simplest
  Sum : Sum  Inputs=|++  SaturateOnIntegerOverflow=on
  guarantee : Outport  OutDataTypeStr=boolean
  wires:
  Relational Operator/1 -> guarantee/1
  output/1 -> Relational Operator/1
  input/1 -> Sum/1
  Sum/1 -> Relational Operator/2
  input1/1 -> Sum/2
